simulink model "SF049A_LoaMgr"  (R2013b)
settings: Solver=FixedStepDiscrete  SolverMode=SingleTasking  StartTime=0.0  StopTime=1  FixedStep=0.002  RelTol=1e-3
values from neighbouring files (symbols this model uses):
  CURRMEASLOAMTGTNMASK_CNT_U08 = DataDict.Constant    [SF049A_LoaMgr_DataDict.m]
  IVTRLOAMTGTNMASK_CNT_U08 = DataDict.Constant    [SF049A_LoaMgr_DataDict.m]
  LOAMAXSLEW_ULSPERSEC_F32 = DataDict.Constant    [SF049A_LoaMgr_DataDict.m]
  LoaMgrCurrIvtrMtgtnRate = DataDict.Calibration    [SF049A_LoaMgr_DataDict.m]
  LoaMgrCurrIvtrMtgtnSca = DataDict.Calibration    [SF049A_LoaMgr_DataDict.m]
  LoaMgrCurrIvtrMtgtnScaZeroEna = DataDict.Calibration    [SF049A_LoaMgr_DataDict.m]
  LoaMgrCurrMeasIdptSig0Resp = DataDict.Calibration    [SF049A_LoaMgr_DataDict.m]
  LoaMgrCurrMeasIdptSig1Resp = DataDict.Calibration    [SF049A_LoaMgr_DataDict.m]
  LoaMgrCurrMeasIdptSig2Resp = DataDict.Calibration    [SF049A_LoaMgr_DataDict.m]
  LoaMgrCurrMeasIdptSigFltThd = DataDict.Calibration    [SF049A_LoaMgr_DataDict.m]
  LoaMgrCurrMeasMtgtnRate = DataDict.Calibration    [SF049A_LoaMgr_DataDict.m]
  LoaMgrCurrMeasMtgtnSca = DataDict.Calibration    [SF049A_LoaMgr_DataDict.m]
  LoaMgrCurrMeasMtgtnScaZeroEna = DataDict.Calibration    [SF049A_LoaMgr_DataDict.m]
  LoaMgrFadeOutStRate = DataDict.Calibration    [SF049A_LoaMgr_DataDict.m]
  LoaMgrHwTqIdptSig0NoTqLoaResp = DataDict.Calibration    [SF049A_LoaMgr_DataDict.m]
  LoaMgrHwTqIdptSig1NoTqLoaResp = DataDict.Calibration    [SF049A_LoaMgr_DataDict.m]
  LoaMgrHwTqIdptSig2Resp = DataDict.Calibration    [SF049A_LoaMgr_DataDict.m]
  LoaMgrHwTqIdptSig4Resp = DataDict.Calibration    [SF049A_LoaMgr_DataDict.m]
  LoaMgrHwTqIdptSigFltThd = DataDict.Calibration    [SF049A_LoaMgr_DataDict.m]
  LoaMgrHwTqLoaAvlResp = DataDict.Calibration    [SF049A_LoaMgr_DataDict.m]
  LoaMgrIvtrIdptSig0Resp = DataDict.Calibration    [SF049A_LoaMgr_DataDict.m]
  LoaMgrIvtrIdptSig1Resp = DataDict.Calibration    [SF049A_LoaMgr_DataDict.m]
  LoaMgrIvtrIdptSig2Resp = DataDict.Calibration    [SF049A_LoaMgr_DataDict.m]
  LoaMgrIvtrIdptSigFltThd = DataDict.Calibration    [SF049A_LoaMgr_DataDict.m]
  LoaMgrIvtrMtgtnRate = DataDict.Calibration    [SF049A_LoaMgr_DataDict.m]
  LoaMgrIvtrMtgtnSca = DataDict.Calibration    [SF049A_LoaMgr_DataDict.m]
  LoaMgrIvtrMtgtnScaZeroEna = DataDict.Calibration    [SF049A_LoaMgr_DataDict.m]
  LoaMgrLimdStRate = DataDict.Calibration    [SF049A_LoaMgr_DataDict.m]
  LoaMgrLimdStSca = DataDict.Calibration    [SF049A_LoaMgr_DataDict.m]
  LoaMgrMotAgAvlSnsrlsResp = DataDict.Calibration    [SF049A_LoaMgr_DataDict.m]
  LoaMgrMotAgIdptSig0NoSnsrlsResp = DataDict.Calibration    [SF049A_LoaMgr_DataDict.m]
  LoaMgrMotAgIdptSig1NoSnsrlsResp = DataDict.Calibration    [SF049A_LoaMgr_DataDict.m]
  LoaMgrMotAgIdptSig2Resp = DataDict.Calibration    [SF049A_LoaMgr_DataDict.m]
  LoaMgrMotAgIdptSig3Resp = DataDict.Calibration    [SF049A_LoaMgr_DataDict.m]
  LoaMgrMotAgIdptSigFltThd = DataDict.Calibration    [SF049A_LoaMgr_DataDict.m]
  LoaMgrMotAgMtgtnRate = DataDict.Calibration    [SF049A_LoaMgr_DataDict.m]
  LoaMgrMotAgMtgtnSca = DataDict.Calibration    [SF049A_LoaMgr_DataDict.m]
  LoaMgrMotAgMtgtnScaZeroEna = DataDict.Calibration    [SF049A_LoaMgr_DataDict.m]
  LOASCAONE_ULS_F32 = DataDict.Constant    [SF049A_LoaMgr_DataDict.m]
  LOASCAZERO_ULS_F32 = DataDict.Constant    [SF049A_LoaMgr_DataDict.m]
  LOASTIMDTSHTDWN_CNT_U08 = DataDict.Constant    [SF049A_LoaMgr_DataDict.m]
  LOASTNORM_CNT_U08 = DataDict.Constant    [SF049A_LoaMgr_DataDict.m]
  LOASTSWMTGTN_CNT_U08 = DataDict.Constant    [SF049A_LoaMgr_DataDict.m]
  MAXCURRMEASIDPTSIGALLWD_CNT_U08 = DataDict.Constant    [SF049A_LoaMgr_DataDict.m]
  MAXHWTQIDPTSIGALLWD_CNT_U08 = DataDict.Constant    [SF049A_LoaMgr_DataDict.m]
  MAXIVTRIDPTSIGALLWD_CNT_U08 = DataDict.Constant    [SF049A_LoaMgr_DataDict.m]
  MAXMOTAGMECLIDPTSIGALLWD_CNT_U08 = DataDict.Constant    [SF049A_LoaMgr_DataDict.m]
  NODEBSTEP_CNT_U16 = DataDict.Constant    [SF049A_LoaMgr_DataDict.m]
undefined symbols (not defined in the file or in its folder): LoaSt1, NtcNr1, NtcSts1, SigQlfr1
libraries: simulink x43, NxtrMin x4, NxtrMax x4, NxtrLim x2
(part 2 of 8)

== system SF049A_LoaMgr/ISO Fault Debounce/DiagMgr/NTCSTS_PREPASSD ==
  EA : Inport
  DS : Inport  Port=2
  TS : Inport  Port=3
  Qlf : Inport  Port=4
  Action Port : ActionPort  ActionType=case
  CopyRight2 : Subsystem  Description=|  mask(Copyright Information){none=on}
      | Copyright info block.                                               
      |                                                                     
      | Place copyright information at the top of every subsystem in design.
      mask prompts: none "No parameters"
      mask help: Place copyright information at the top of every subsystem in design.
      mask Display:
      | NxtrConf = 'Nexteer Confidential';
      | 
      | sys = bdroot; %handle for the current model ("system")
      | first = get_param(sys,'Created');
      | first = first(end-3:end);  %year is last four digits
      | 
      | last = get_param(sys,'LastModifiedDate');
      | if isempty(last)
      |     last = datestr(now,'yyyy');
      | else
      |     last = last(end-3:end);
      | end
      | 
      | if strcmp(first,last)
      |     fprintf('%s -- Copyright %s Nexteer',NxtrConf,first)
      | else
      |     fprintf('%s -- %s%s- %s Nexteer',NxtrConf,char(169),first,last)
      | end
  If : If  NumInputs=2  IfExpression=u1 <= u2
  If Action Subsystem : Subsystem  TreatAsAtomicUnit=on
  If Action Subsystem1 : Subsystem  TreatAsAtomicUnit=on
  Merge : Merge
  Merge1 : Merge
  QlfPassd : Constant  Value=SigQlfr1.SIGQLFR_PASSD  OutDataTypeStr=Enum: SigQlfr1
  Sum : Sum  Inputs=|+-
  Unary Minus : UnaryMinus
  EAo : Outport
  Qlfo : Outport  Port=2
  wires:
  EA/1 -> Sum/1
  DS/1 -> Sum/2
  Sum/1 -> If Action Subsystem1/1(In1), If/1
  TS/1 -> [Threshold], If/2
  If/1 -> If Action Subsystem/Action
  Unary Minus/1 -> If Action Subsystem/1(In1)
  If Action Subsystem/1(Out1) -> Merge/1
  If Action Subsystem1/1(Out1) -> Merge/2
  Merge/1 -> EAo/1
  If Action Subsystem/2(Out2) -> Merge1/1
  If Action Subsystem1/2(Out2) -> Merge1/2
  Merge1/1 -> Qlfo/1
  QlfPassd/1 -> If Action Subsystem/2(In2)
  Qlf/1 -> If Action Subsystem1/2(In2)
  If/2 -> If Action Subsystem1/Action
  [Threshold] -> Unary Minus/1

== system SF049A_LoaMgr/ISO Fault Debounce/DiagMgr/Set Latch ==
  In1 : Inport
  Action Port : ActionPort  ActionType=then
  Out1 : Outport
  wires:
  In1/1 -> Out1/1

== system SF049A_LoaMgr/LoaMgr/LoaMgrInit1/CopyRight2 ==

== system SF049A_LoaMgr/LoaMgr/LoaMgrInit1/NTC_Fault1 ==
  NtcNr : Inport
  NtcStInfo : Inport  Port=2
  NtcSts : Inport  Port=3
  DebStep : Inport  Port=4
  SetNtcSts : Subsystem  RequirementInfo={} %GIDa_23fdb935_d0cd_490e_ba1d_400dad3b5aaf  TreatAsAtomicUnit=on
      settings: RTWSystemCode=Inline
  wires:
  NtcNr/1 -> SetNtcSts/1(NtcNr)  "NtcNr"
  NtcSts/1 -> SetNtcSts/3(NtcSts)
  DebStep/1 -> SetNtcSts/4(DebStep)
  NtcStInfo/1 -> SetNtcSts/2(NtcStInfo)

== system SF049A_LoaMgr/LoaMgr/LoaMgrInit1/NTC_Fault2 ==
  NtcNr : Inport
  NtcStInfo : Inport  Port=2
  NtcSts : Inport  Port=3
  DebStep : Inport  Port=4
  SetNtcSts : Subsystem  RequirementInfo={} %GIDa_89eb5662_1adb_446a_ae4b_e7f3c6b102b6  TreatAsAtomicUnit=on
      settings: RTWSystemCode=Inline
  wires:
  NtcStInfo/1 -> SetNtcSts/2(NtcStInfo)
  DebStep/1 -> SetNtcSts/4(DebStep)
  NtcSts/1 -> SetNtcSts/3(NtcSts)
  NtcNr/1 -> SetNtcSts/1(NtcNr)  "NtcNr"

== system SF049A_LoaMgr/LoaMgr/LoaMgrInit1/NTC_Fault3 ==
  NtcNr : Inport
  NtcStInfo : Inport  Port=2
  NtcSts : Inport  Port=3
  DebStep : Inport  Port=4
  SetNtcSts : Subsystem  RequirementInfo={} %GIDa_2736ae0d_ecf6_416e_8429_36e35a164155  TreatAsAtomicUnit=on
      settings: RTWSystemCode=Inline
  wires:
  NtcStInfo/1 -> SetNtcSts/2(NtcStInfo)
  DebStep/1 -> SetNtcSts/4(DebStep)
  NtcSts/1 -> SetNtcSts/3(NtcSts)
  NtcNr/1 -> SetNtcSts/1(NtcNr)  "NtcNr"

== system SF049A_LoaMgr/LoaMgr/LoaMgrInit1/NTC_Fault4 ==
  NtcNr : Inport
  NtcStInfo : Inport  Port=2
  NtcSts : Inport  Port=3
  DebStep : Inport  Port=4
  SetNtcSts : Subsystem  RequirementInfo={} %GIDa_c84246ca_06da_45c0_bfee_0800e0212aeb  TreatAsAtomicUnit=on
      settings: RTWSystemCode=Inline
  wires:
  NtcNr/1 -> SetNtcSts/1(NtcNr)  "NtcNr"
  NtcSts/1 -> SetNtcSts/3(NtcSts)
  DebStep/1 -> SetNtcSts/4(DebStep)
  NtcStInfo/1 -> SetNtcSts/2(NtcStInfo)

== system SF049A_LoaMgr/LoaMgr/LoaMgrInit1/NTC_Fault5 ==
  NtcNr : Inport
  NtcStInfo : Inport  Port=2
  NtcSts : Inport  Port=3
  DebStep : Inport  Port=4
  SetNtcSts : Subsystem  RequirementInfo={} %GIDa_5e8c2de6_0cb9_44b1_8719_e4221f2f855f  TreatAsAtomicUnit=on
      settings: RTWSystemCode=Inline
  wires:
  NtcStInfo/1 -> SetNtcSts/2(NtcStInfo)
  DebStep/1 -> SetNtcSts/4(DebStep)
  NtcSts/1 -> SetNtcSts/3(NtcSts)
  NtcNr/1 -> SetNtcSts/1(NtcNr)  "NtcNr"

== system SF049A_LoaMgr/LoaMgr/LoaMgrInit1/NTC_Fault6 ==
  NtcNr : Inport
  NtcStInfo : Inport  Port=2
  NtcSts : Inport  Port=3
  DebStep : Inport  Port=4
  SetNtcSts : Subsystem  RequirementInfo={} %GIDa_1fd4e5c0_5e97_4c72_b752_8c7dcd130455  TreatAsAtomicUnit=on
      settings: RTWSystemCode=Inline
  wires:
  NtcStInfo/1 -> SetNtcSts/2(NtcStInfo)
  DebStep/1 -> SetNtcSts/4(DebStep)
  NtcSts/1 -> SetNtcSts/3(NtcSts)
  NtcNr/1 -> SetNtcSts/1(NtcNr)  "NtcNr"

== system SF049A_LoaMgr/LoaMgr/LoaMgrPer1/Arbitrate_Responses ==
  note: Individual responses can set boolean flags to true to direct downstream functions.
      | The combination of individual responses generates its own "multiple mitigation response".
      | The final LoaState response will be the worst case of individual and "multiple mitigation" responses.
  RespMux : Inport
  CntSwBasdMtgtn : Subsystem
  CopyRight2 : Subsystem  Description=|  mask(Copyright Information){none=on}
      | Copyright info block.                                               
      |                                                                     
      | Place copyright information at the top of every subsystem in design.
      mask prompts: none "No parameters"
      mask help: Place copyright information at the top of every subsystem in design.
      mask Display:
      | NxtrConf = 'Nexteer Confidential';
      | 
      | sys = bdroot; %handle for the current model ("system")
      | first = get_param(sys,'Created');
      | first = first(end-3:end);  %year is last four digits
      | 
      | last = get_param(sys,'LastModifiedDate');
      | if isempty(last)
      |     last = datestr(now,'yyyy');
      | else
      |     last = last(end-3:end);
      | end
      | 
      | if strcmp(first,last)
      |     fprintf('%s -- Copyright %s Nexteer',NxtrConf,first)
      | else
      |     fprintf('%s -- %s%s- %s Nexteer',NxtrConf,char(169),first,last)
      | end
  Demux : Demux
  Demux1 : Demux
  Mux : Mux
  SelFinalResp : Subsystem
  LoaState : Outport  RequirementInfo="{'linktype_rmi_doors' '0000bab3 (/E-STEER Core/SubSystem Specifications/Application Functions/SF049A Loss of Assist Manager)' '#SF049A_84' 'true' 'REQ:  SF049A_84' '' } %GIDa_2917bb2b_4bd4_4079_ac09_4ef15e442a03"
  SwMtgtnEnMux : Outport  Port=2
  wires:
  Demux/1 -> CntSwBasdMtgtn/1(HwTqResp)
  Demux/2 -> CntSwBasdMtgtn/2(MotAgResp)
  Demux/3 -> CntSwBasdMtgtn/3(CurrMeasResp)
  Demux/4 -> CntSwBasdMtgtn/4(IvtrResp)
  CntSwBasdMtgtn/1(HwTqLoaMtgtnEna) -> Mux/1  "HwTqLoaMtgtnEna"
  CntSwBasdMtgtn/2(MotAgLoaMtgtnEna) -> Mux/2  "MotAgLoaMtgtnEna"
  CntSwBasdMtgtn/3(CurrMeasLoaMtgtnEna) -> Mux/3  "CurrMeasLoaMtgtnEna"
  CntSwBasdMtgtn/4(IvtrLoaMtgtnEna) -> Mux/4  "IvtrLoaMtgtnEna"
  Mux/1 -> SwMtgtnEnMux/1
  CntSwBasdMtgtn/5(MultiMtgtnResp) -> SelFinalResp/1(MultiMtgtnResp)
  RespMux/1 -> Demux1/1, Demux/1
  Demux1/1 -> SelFinalResp/2(HwTqResp)
  Demux1/2 -> SelFinalResp/3(MotAgResp)
  Demux1/3 -> SelFinalResp/4(CurrMeasResp)
  Demux1/4 -> SelFinalResp/5(IvtrResp)
  SelFinalResp/1(LoaSt) -> LoaState/1

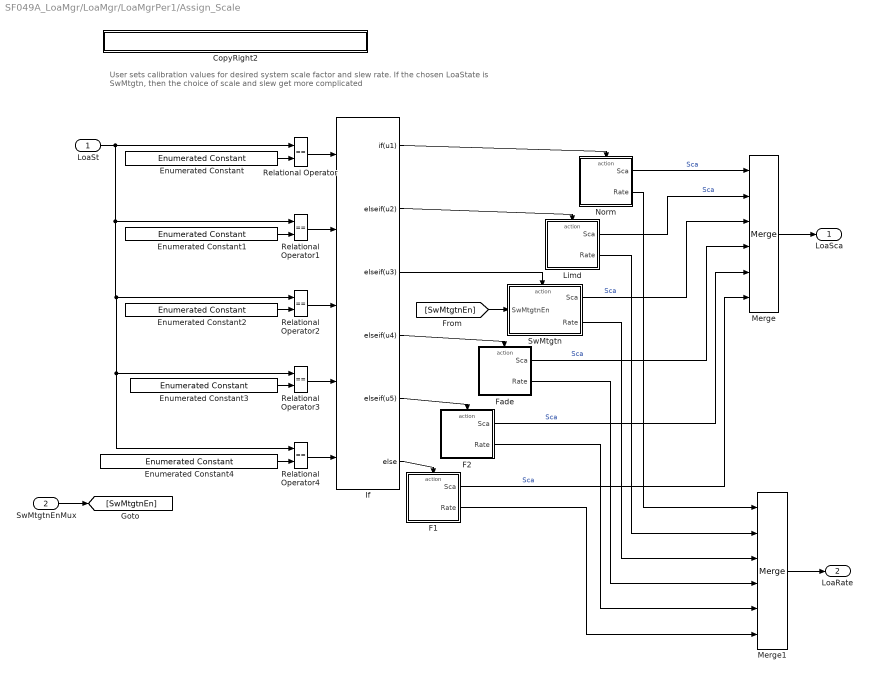
== system SF049A_LoaMgr/LoaMgr/LoaMgrPer1/Assign_Scale ==
  note: User sets calibration values for desired system scale factor and slew rate.  If the chosen LoaState is SwMtgtn, then the choice of
      | scale and slew get more complicated
  LoaSt : Inport  RequirementInfo="{'linktype_rmi_doors' '0000bab3 (/E-STEER Core/SubSystem Specifications/Application Functions/SF049A Loss of Assist Manager)' '#SF049A_93' 'true' 'REQ:  SF049A_93' '' ; 'linktype_rmi_doors' '0000bab3 (/E-STEER Core/SubSystem Specifications/Application Functions/SF049A Loss of Assist Manager)' '#SF049A_94' 'true' 'REQ:  SF049A_94' '' ; 'linktype_rmi_doors' '0000bab3 (/E-STEER Core/SubSystem Specifications/Application Functions/SF049A Loss of Assist Manager)' '#SF049A_95' 'true' 'REQ:  SF049A_95' '' ; 'linktype_rmi_doors' '0000bab3 (/E-STEER Core/SubSystem Specifications/Application Functions/SF049A Loss of Assist Manager)' '#SF049A_96' 'true' 'REQ:  SF049A_96' '' ; 'linktype_rmi_doors' '0000bab3 (/E-STEER Core/SubSystem Specifications/Application Functions/SF049A Loss of Assist Manager)' '#SF049A_97' 'true' 'REQ:  SF049A_97' '' ; 'linktype_rmi_doors' '0000bab3 (/E-STEER Core/SubSystem Specifications/Application Functions/SF049A Loss of Assist Manager)' '#SF049A_100' 'true' 'REQ:  SF049A_100' '' } %GIDa_3e7875f7_b2dd_4b11_87a2_7c0344e13c7b"
  SwMtgtnEnMux : Inport  RequirementInfo="{'linktype_rmi_doors' '0000bab3 (/E-STEER Core/SubSystem Specifications/Application Functions/SF049A Loss of Assist Manager)' '#SF049A_99' 'true' 'REQ:  SF049A_99' '' ; 'linktype_rmi_doors' '0000bab3 (/E-STEER Core/SubSystem Specifications/Application Functions/SF049A Loss of Assist Manager)' '#SF049A_100' 'true' 'REQ:  SF049A_100' '' } %GIDa_9818a3a5_64db_45b2_8dab_2de682de8c50"  Port=2
  CopyRight2 : Subsystem  Description=|  mask(Copyright Information){none=on}
      | Copyright info block.                                               
      |                                                                     
      | Place copyright information at the top of every subsystem in design.
      mask prompts: none "No parameters"
      mask help: Place copyright information at the top of every subsystem in design.
      mask Display:
      | NxtrConf = 'Nexteer Confidential';
      | 
      | sys = bdroot; %handle for the current model ("system")
      | first = get_param(sys,'Created');
      | first = first(end-3:end);  %year is last four digits
      | 
      | last = get_param(sys,'LastModifiedDate');
      | if isempty(last)
      |     last = datestr(now,'yyyy');
      | else
      |     last = last(end-3:end);
      | end
      | 
      | if strcmp(first,last)
      |     fprintf('%s -- Copyright %s Nexteer',NxtrConf,first)
      | else
      |     fprintf('%s -- %s%s- %s Nexteer',NxtrConf,char(169),first,last)
      | end
  Enumerated Constant : simulink/Sources/Enumerated Constant  RequirementInfo="{'linktype_rmi_doors' '0000bab3 (/E-STEER Core/SubSystem Specifications/Application Functions/SF049A Loss of Assist Manager)' '#SF049A_93' 'true' 'REQ:  SF049A_93' '' } %GIDa_f27a0b99_a290_4ea5_abd7_4a8bd3123567"  OutDataTypeStr=Enum: LoaSt1  Value=LoaSt1.LOAST_NORM  SampleTime=inf
  Enumerated Constant1 : simulink/Sources/Enumerated Constant  RequirementInfo="{'linktype_rmi_doors' '0000bab3 (/E-STEER Core/SubSystem Specifications/Application Functions/SF049A Loss of Assist Manager)' '#SF049A_94' 'true' 'REQ:  SF049A_94' '' } %GIDa_d920381e_876a_4e76_93ae_b2656d59d1b0"  OutDataTypeStr=Enum: LoaSt1  Value=LoaSt1.LOAST_LIMD  SampleTime=inf
  Enumerated Constant2 : simulink/Sources/Enumerated Constant  RequirementInfo="{'linktype_rmi_doors' '0000bab3 (/E-STEER Core/SubSystem Specifications/Application Functions/SF049A Loss of Assist Manager)' '#SF049A_99' 'true' 'REQ:  SF049A_99' '' ; 'linktype_rmi_doors' '0000bab3 (/E-STEER Core/SubSystem Specifications/Application Functions/SF049A Loss of Assist Manager)' '#SF049A_100' 'true' 'REQ:  SF049A_100' '' } %GIDa_83a64fdd_b2aa_4bd7_b652_9878089e09b4"  OutDataTypeStr=Enum: LoaSt1  Value=LoaSt1.LOAST_SWBASDMTGTN  SampleTime=inf
  Enumerated Constant3 : simulink/Sources/Enumerated Constant  RequirementInfo="{'linktype_rmi_doors' '0000bab3 (/E-STEER Core/SubSystem Specifications/Application Functions/SF049A Loss of Assist Manager)' '#SF049A_95' 'true' 'REQ:  SF049A_95' '' } %GIDa_647ea362_d5ca_4b6a_9517_1cd75c76e2d9"  OutDataTypeStr=Enum: LoaSt1  Value=LoaSt1.LOAST_FADEOUT  SampleTime=inf
  Enumerated Constant4 : simulink/Sources/Enumerated Constant  RequirementInfo="{'linktype_rmi_doors' '0000bab3 (/E-STEER Core/SubSystem Specifications/Application Functions/SF049A Loss of Assist Manager)' '#SF049A_96' 'true' 'REQ:  SF049A_96' '' } %GIDa_cd78f97b_5efc_4e4a_8ad5_30890b04384b"  OutDataTypeStr=Enum: LoaSt1  Value=LoaSt1.LOAST_CTRLDSHTDWNREQD  SampleTime=inf
  F1 : Subsystem  RequirementInfo="{'linktype_rmi_doors' '0000bab3 (/E-STEER Core/SubSystem Specifications/Application Functions/SF049A Loss of Assist Manager)' '#SF049A_97' 'true' 'REQ:  SF049A_97' '' } %GIDa_e1aaa04d_b9cf_4590_9790_e96624afa4aa"  TreatAsAtomicUnit=on
      settings: RTWSystemCode=Inline
  F2 : Subsystem  RequirementInfo="{'linktype_rmi_doors' '0000bab3 (/E-STEER Core/SubSystem Specifications/Application Functions/SF049A Loss of Assist Manager)' '#SF049A_96' 'true' 'REQ:  SF049A_96' '' } %GIDa_1938d1a4_6ea2_4bb3_af5e_d31a0fe8b378"  TreatAsAtomicUnit=on
      settings: RTWSystemCode=Inline
  Fade : Subsystem  RequirementInfo="{'linktype_rmi_doors' '0000bab3 (/E-STEER Core/SubSystem Specifications/Application Functions/SF049A Loss of Assist Manager)' '#SF049A_95' 'true' 'REQ:  SF049A_95' '' } %GIDa_5c4662ce_ee53_4f4f_ae03_f1d5fbfaeef4"  TreatAsAtomicUnit=on
      settings: RTWSystemCode=Inline
  If : If  RequirementInfo="{'linktype_rmi_doors' '0000bab3 (/E-STEER Core/SubSystem Specifications/Application Functions/SF049A Loss of Assist Manager)' '#SF049A_93' 'true' 'REQ:  SF049A_93' '' ; 'linktype_rmi_doors' '0000bab3 (/E-STEER Core/SubSystem Specifications/Application Functions/SF049A Loss of Assist Manager)' '#SF049A_94' 'true' 'REQ:  SF049A_94' '' ; 'linktype_rmi_doors' '0000bab3 (/E-STEER Core/SubSystem Specifications/Application Functions/SF049A Loss of Assist Manager)' '#SF049A_95' 'true' 'REQ:  SF049A_95' '' ; 'linktype_rmi_doors' '0000bab3 (/E-STEER Core/SubSystem Specifications/Application Functions/SF049A Loss of Assist Manager)' '#SF049A_96' 'true' 'REQ:  SF049A_96' '' ; 'linktype_rmi_doors' '0000bab3 (/E-STEER Core/SubSystem Specifications/Application Functions/SF049A Loss of Assist Manager)' '#SF049A_97' 'true' 'REQ:  SF049A_97' '' ; 'linktype_rmi_doors' '0000bab3 (/E-STEER Core/SubSystem Specifications/Application Functions/SF049A Loss of Assist Manager)' '#SF049A_99' 'true' 'REQ:  SF049A_99' '' ; 'linktype_rmi_doors' '0000bab3 (/E-STEER Core/SubSystem Specifications/Application Functions/SF049A Loss of Assist Manager)' '#SF049A_100' 'true' 'REQ:  SF049A_100' '' } %GIDa_5c51bdba_2274_48ad_8412_9716f3180cc7"  NumInputs=5  IfExpression=u1  ElseIfExpressions=u2, u3,u4,u5
  Limd : Subsystem  RequirementInfo="{'linktype_rmi_doors' '0000bab3 (/E-STEER Core/SubSystem Specifications/Application Functions/SF049A Loss of Assist Manager)' '#SF049A_94' 'true' 'REQ:  SF049A_94' '' } %GIDa_f0a5710c_890a_4ef1_b79a_7c37771acf89"  TreatAsAtomicUnit=on
      settings: RTWSystemCode=Inline
  Merge : Merge  RequirementInfo="{'linktype_rmi_doors' '0000bab3 (/E-STEER Core/SubSystem Specifications/Application Functions/SF049A Loss of Assist Manager)' '#SF049A_93' 'true' 'REQ:  SF049A_93' '' ; 'linktype_rmi_doors' '0000bab3 (/E-STEER Core/SubSystem Specifications/Application Functions/SF049A Loss of Assist Manager)' '#SF049A_94' 'true' 'REQ:  SF049A_94' '' ; 'linktype_rmi_doors' '0000bab3 (/E-STEER Core/SubSystem Specifications/Application Functions/SF049A Loss of Assist Manager)' '#SF049A_95' 'true' 'REQ:  SF049A_95' '' ; 'linktype_rmi_doors' '0000bab3 (/E-STEER Core/SubSystem Specifications/Application Functions/SF049A Loss of Assist Manager)' '#SF049A_96' 'true' 'REQ:  SF049A_96' '' ; 'linktype_rmi_doors' '0000bab3 (/E-STEER Core/SubSystem Specifications/Application Functions/SF049A Loss of Assist Manager)' '#SF049A_97' 'true' 'REQ:  SF049A_97' '' ; 'linktype_rmi_doors' '0000bab3 (/E-STEER Core/SubSystem Specifications/Application Functions/SF049A Loss of Assist Manager)' '#SF049A_99' 'true' 'REQ:  SF049A_99' '' ; 'linktype_rmi_doors' '0000bab3 (/E-STEER Core/SubSystem Specifications/Application Functions/SF049A Loss of Assist Manager)' '#SF049A_100' 'true' 'REQ:  SF049A_100' '' } %GIDa_3b299f34_e795_470f_ac90_16d0d3d510be"  Inputs=6
  Merge1 : Merge  RequirementInfo="{'linktype_rmi_doors' '0000bab3 (/E-STEER Core/SubSystem Specifications/Application Functions/SF049A Loss of Assist Manager)' '#SF049A_93' 'true' 'REQ:  SF049A_93' '' ; 'linktype_rmi_doors' '0000bab3 (/E-STEER Core/SubSystem Specifications/Application Functions/SF049A Loss of Assist Manager)' '#SF049A_94' 'true' 'REQ:  SF049A_94' '' ; 'linktype_rmi_doors' '0000bab3 (/E-STEER Core/SubSystem Specifications/Application Functions/SF049A Loss of Assist Manager)' '#SF049A_95' 'true' 'REQ:  SF049A_95' '' ; 'linktype_rmi_doors' '0000bab3 (/E-STEER Core/SubSystem Specifications/Application Functions/SF049A Loss of Assist Manager)' '#SF049A_96' 'true' 'REQ:  SF049A_96' '' ; 'linktype_rmi_doors' '0000bab3 (/E-STEER Core/SubSystem Specifications/Application Functions/SF049A Loss of Assist Manager)' '#SF049A_97' 'true' 'REQ:  SF049A_97' '' ; 'linktype_rmi_doors' '0000bab3 (/E-STEER Core/SubSystem Specifications/Application Functions/SF049A Loss of Assist Manager)' '#SF049A_99' 'true' 'REQ:  SF049A_99' '' ; 'linktype_rmi_doors' '0000bab3 (/E-STEER Core/SubSystem Specifications/Application Functions/SF049A Loss of Assist Manager)' '#SF049A_100' 'true' 'REQ:  SF049A_100' '' } %GIDa_74c15a35_1fbd_4169_b897_3cf740b201ea"  Inputs=6
  Norm : Subsystem  RequirementInfo="{'linktype_rmi_doors' '0000bab3 (/E-STEER Core/SubSystem Specifications/Application Functions/SF049A Loss of Assist Manager)' '#SF049A_93' 'true' 'REQ:  SF049A_93' '' } %GIDa_c9df33ca_5dd7_489e_a91a_aa4b767aa5db"  TreatAsAtomicUnit=on
      settings: RTWSystemCode=Inline
  Relational Operator : RelationalOperator  RequirementInfo="{'linktype_rmi_doors' '0000bab3 (/E-STEER Core/SubSystem Specifications/Application Functions/SF049A Loss of Assist Manager)' '#SF049A_93' 'true' 'REQ:  SF049A_93' '' } %GIDa_da08ce41_39bd_4e01_b620_6f9860489864"  Operator===  OutDataTypeStr=boolean
  Relational Operator1 : RelationalOperator  RequirementInfo="{'linktype_rmi_doors' '0000bab3 (/E-STEER Core/SubSystem Specifications/Application Functions/SF049A Loss of Assist Manager)' '#SF049A_94' 'true' 'REQ:  SF049A_94' '' } %GIDa_10d94627_2d94_4d9c_8055_2d3addac56cd"  Operator===  OutDataTypeStr=boolean
  Relational Operator2 : RelationalOperator  RequirementInfo="{'linktype_rmi_doors' '0000bab3 (/E-STEER Core/SubSystem Specifications/Application Functions/SF049A Loss of Assist Manager)' '#SF049A_99' 'true' 'REQ:  SF049A_99' '' ; 'linktype_rmi_doors' '0000bab3 (/E-STEER Core/SubSystem Specifications/Application Functions/SF049A Loss of Assist Manager)' '#SF049A_100' 'true' 'REQ:  SF049A_100' '' } %GIDa_6fb469fc_d1b3_4ed9_bf7f_ce037c3366d3"  Operator===  OutDataTypeStr=boolean
  Relational Operator3 : RelationalOperator  RequirementInfo="{'linktype_rmi_doors' '0000bab3 (/E-STEER Core/SubSystem Specifications/Application Functions/SF049A Loss of Assist Manager)' '#SF049A_95' 'true' 'REQ:  SF049A_95' '' } %GIDa_85f97dac_396b_438a_bfaa_297eb3998244"  Operator===  OutDataTypeStr=boolean
  Relational Operator4 : RelationalOperator  RequirementInfo="{'linktype_rmi_doors' '0000bab3 (/E-STEER Core/SubSystem Specifications/Application Functions/SF049A Loss of Assist Manager)' '#SF049A_96' 'true' 'REQ:  SF049A_96' '' } %GIDa_ea11fa20_b626_4bfa_a544_554563d25da6"  Operator===  OutDataTypeStr=boolean
  SwMtgtn : Subsystem  RequirementInfo="{'linktype_rmi_doors' '0000bab3 (/E-STEER Core/SubSystem Specifications/Application Functions/SF049A Loss of Assist Manager)' '#SF049A_99' 'true' 'REQ:  SF049A_99' '' ; 'linktype_rmi_doors' '0000bab3 (/E-STEER Core/SubSystem Specifications/Application Functions/SF049A Loss of Assist Manager)' '#SF049A_100' 'true' 'REQ:  SF049A_100' '' } %GIDa_0f2bff9a_81bf_40ef_b624_524280b34e28"  TreatAsAtomicUnit=on
      settings: RTWSystemCode=Inline
  LoaSca : Outport  RequirementInfo="{'linktype_rmi_doors' '0000bab3 (/E-STEER Core/SubSystem Specifications/Application Functions/SF049A Loss of Assist Manager)' '#SF049A_93' 'true' 'REQ:  SF049A_93' '' ; 'linktype_rmi_doors' '0000bab3 (/E-STEER Core/SubSystem Specifications/Application Functions/SF049A Loss of Assist Manager)' '#SF049A_94' 'true' 'REQ:  SF049A_94' '' ; 'linktype_rmi_doors' '0000bab3 (/E-STEER Core/SubSystem Specifications/Application Functions/SF049A Loss of Assist Manager)' '#SF049A_95' 'true' 'REQ:  SF049A_95' '' ; 'linktype_rmi_doors' '0000bab3 (/E-STEER Core/SubSystem Specifications/Application Functions/SF049A Loss of Assist Manager)' '#SF049A_96' 'true' 'REQ:  SF049A_96' '' ; 'linktype_rmi_doors' '0000bab3 (/E-STEER Core/SubSystem Specifications/Application Functions/SF049A Loss of Assist Manager)' '#SF049A_97' 'true' 'REQ:  SF049A_97' '' ; 'linktype_rmi_doors' '0000bab3 (/E-STEER Core/SubSystem Specifications/Application Functions/SF049A Loss of Assist Manager)' '#SF049A_99' 'true' 'REQ:  SF049A_99' '' ; 'linktype_rmi_doors' '0000bab3 (/E-STEER Core/SubSystem Specifications/Application Functions/SF049A Loss of Assist Manager)' '#SF049A_100' 'true' 'REQ:  SF049A_100' '' } %GIDa_169a2149_2e31_4d28_bbf1_074d98108588"
  LoaRate : Outport  RequirementInfo="{'linktype_rmi_doors' '0000bab3 (/E-STEER Core/SubSystem Specifications/Application Functions/SF049A Loss of Assist Manager)' '#SF049A_93' 'true' 'REQ:  SF049A_93' '' ; 'linktype_rmi_doors' '0000bab3 (/E-STEER Core/SubSystem Specifications/Application Functions/SF049A Loss of Assist Manager)' '#SF049A_94' 'true' 'REQ:  SF049A_94' '' ; 'linktype_rmi_doors' '0000bab3 (/E-STEER Core/SubSystem Specifications/Application Functions/SF049A Loss of Assist Manager)' '#SF049A_95' 'true' 'REQ:  SF049A_95' '' ; 'linktype_rmi_doors' '0000bab3 (/E-STEER Core/SubSystem Specifications/Application Functions/SF049A Loss of Assist Manager)' '#SF049A_96' 'true' 'REQ:  SF049A_96' '' ; 'linktype_rmi_doors' '0000bab3 (/E-STEER Core/SubSystem Specifications/Application Functions/SF049A Loss of Assist Manager)' '#SF049A_97' 'true' 'REQ:  SF049A_97' '' ; 'linktype_rmi_doors' '0000bab3 (/E-STEER Core/SubSystem Specifications/Application Functions/SF049A Loss of Assist Manager)' '#SF049A_99' 'true' 'REQ:  SF049A_99' '' ; 'linktype_rmi_doors' '0000bab3 (/E-STEER Core/SubSystem Specifications/Application Functions/SF049A Loss of Assist Manager)' '#SF049A_100' 'true' 'REQ:  SF049A_100' '' } %GIDa_8cb2e7f7_efc3_4bfe_b724_767c9179be15"  Port=2
  wires:
  Enumerated Constant/1 -> Relational Operator/2
  Enumerated Constant1/1 -> Relational Operator1/2
  Enumerated Constant2/1 -> Relational Operator2/2
  Enumerated Constant3/1 -> Relational Operator3/2
  LoaSt/1 -> Relational Operator4/1, Relational Operator3/1, Relational Operator2/1, Relational Operator1/1, Relational Operator/1
  Enumerated Constant4/1 -> Relational Operator4/2
  Relational Operator/1 -> If/1
  Relational Operator1/1 -> If/2
  Relational Operator2/1 -> If/3
  Relational Operator3/1 -> If/4
  Relational Operator4/1 -> If/5
  If/1 -> Norm/Action
  If/2 -> Limd/Action
  If/3 -> SwMtgtn/Action
  If/4 -> Fade/Action
  If/5 -> F2/Action
  If/6 -> F1/Action
  Norm/1(Sca) -> Merge/1  "Sca"
  Limd/1(Sca) -> Merge/2  "Sca"
  Fade/1(Sca) -> Merge/4  "Sca"
  F2/1(Sca) -> Merge/5  "Sca"
  F1/1(Sca) -> Merge/6  "Sca"
  Merge/1 -> LoaSca/1
  Norm/2(Rate) -> Merge1/1
  Limd/2(Rate) -> Merge1/2
  Fade/2(Rate) -> Merge1/4
  F2/2(Rate) -> Merge1/5
  F1/2(Rate) -> Merge1/6
  Merge1/1 -> LoaRate/1
  SwMtgtnEnMux/1 -> [SwMtgtnEn]
  [SwMtgtnEn] -> SwMtgtn/1(SwMtgtnEn)
  SwMtgtn/1(Sca) -> Merge/3  "Sca"
  SwMtgtn/2(Rate) -> Merge1/3

== system SF049A_LoaMgr/LoaMgr/LoaMgrPer1/Calc_Ivtr_State ==
  note: Nexter coding standards prevent the casting of boolean signals to other datatypes.
      | If that rule did not exist, this logic would use convert blocks to cast each boolean
      | to uint8, then add them up.
  Ivtr1Inactv : Inport  RequirementInfo="{'linktype_rmi_doors' '0000bab3 (/E-STEER Core/SubSystem Specifications/Application Functions/SF049A Loss of Assist Manager)' '#SF049A_183' 'true' 'REQ:  SF049A_183' '' } %GIDa_de6ec2ea_e682_4d17_b4f6_aabeca528bd3"
  Ivtr2Inactv : Inport  RequirementInfo="{'linktype_rmi_doors' '0000bab3 (/E-STEER Core/SubSystem Specifications/Application Functions/SF049A Loss of Assist Manager)' '#SF049A_183' 'true' 'REQ:  SF049A_183' '' } %GIDa_968df205_4920_4db1_82fc_3b23eb8eeb61"  Port=2
  " " : Merge  RequirementInfo="{'linktype_rmi_doors' '0000bab3 (/E-STEER Core/SubSystem Specifications/Application Functions/SF049A Loss of Assist Manager)' '#SF049A_183' 'true' 'REQ:  SF049A_183' '' } %GIDa_6e820a2a_9d7d_4387_81a9_e3b6b43a99ee"
  " 1" : Merge  RequirementInfo="{'linktype_rmi_doors' '0000bab3 (/E-STEER Core/SubSystem Specifications/Application Functions/SF049A Loss of Assist Manager)' '#SF049A_183' 'true' 'REQ:  SF049A_183' '' } %GIDa_4be40db0_e2f0_494d_962c_150a10a22e37"
  Add1 : Sum  RequirementInfo="{'linktype_rmi_doors' '0000bab3 (/E-STEER Core/SubSystem Specifications/Application Functions/SF049A Loss of Assist Manager)' '#SF049A_183' 'true' 'REQ:  SF049A_183' '' } %GIDa_6635589d_766f_4912_9afd_5eff77041ff3"
  Constant1 : Constant  RequirementInfo="{'linktype_rmi_doors' '0000bab3 (/E-STEER Core/SubSystem Specifications/Application Functions/SF049A Loss of Assist Manager)' '#SF049A_183' 'true' 'REQ:  SF049A_183' '' } %GIDa_41bc2e65_c215_4d13_87d4_1d9f310de0af"  OutDataTypeStr=uint8
      settings: AttributesFormatString=%<OutDataTypeStr>
  Constant2 : Constant  RequirementInfo="{'linktype_rmi_doors' '0000bab3 (/E-STEER Core/SubSystem Specifications/Application Functions/SF049A Loss of Assist Manager)' '#SF049A_183' 'true' 'REQ:  SF049A_183' '' } %GIDa_12d9b86f_40e2_490f_b7b6_b5286bb30cc6"  Value=0  OutDataTypeStr=uint8
      settings: AttributesFormatString=%<OutDataTypeStr>
  Constant4 : Constant  RequirementInfo="{'linktype_rmi_doors' '0000bab3 (/E-STEER Core/SubSystem Specifications/Application Functions/SF049A Loss of Assist Manager)' '#SF049A_183' 'true' 'REQ:  SF049A_183' '' } %GIDa_91ec947b_8597_46f0_9f25_34857e4f337d"  Value=0  OutDataTypeStr=uint8
      settings: AttributesFormatString=%<OutDataTypeStr>
  Constant6 : Constant  RequirementInfo="{'linktype_rmi_doors' '0000bab3 (/E-STEER Core/SubSystem Specifications/Application Functions/SF049A Loss of Assist Manager)' '#SF049A_183' 'true' 'REQ:  SF049A_183' '' } %GIDa_cebea097_c2b2_4a90_91e2_d089833dbd9f"  OutDataTypeStr=uint8
      settings: AttributesFormatString=%<OutDataTypeStr>
  CopyRight2 : Subsystem  Description=|  mask(Copyright Information){none=on}
      | Copyright info block.                                               
      |                                                                     
      | Place copyright information at the top of every subsystem in design.
      mask prompts: none "No parameters"
      mask help: Place copyright information at the top of every subsystem in design.
      mask Display:
      | NxtrConf = 'Nexteer Confidential';
      | 
      | sys = bdroot; %handle for the current model ("system")
      | first = get_param(sys,'Created');
      | first = first(end-3:end);  %year is last four digits
      | 
      | last = get_param(sys,'LastModifiedDate');
      | if isempty(last)
      |     last = datestr(now,'yyyy');
      | else
      |     last = last(end-3:end);
      | end
      | 
      | if strcmp(first,last)
      |     fprintf('%s -- Copyright %s Nexteer',NxtrConf,first)
      | else
      |     fprintf('%s -- %s%s- %s Nexteer',NxtrConf,char(169),first,last)
      | end
  Ivtr1Inactv_IF : If  RequirementInfo="{'linktype_rmi_doors' '0000bab3 (/E-STEER Core/SubSystem Specifications/Application Functions/SF049A Loss of Assist Manager)' '#SF049A_183' 'true' 'REQ:  SF049A_183' '' } %GIDa_1d0fb7e6_1c31_4e80_b36a_c03c6493b93e"  IfExpression=u1
  Ivtr1Sts_ELSE : Subsystem  RequirementInfo="{'linktype_rmi_doors' '0000bab3 (/E-STEER Core/SubSystem Specifications/Application Functions/SF049A Loss of Assist Manager)' '#SF049A_183' 'true' 'REQ:  SF049A_183' '' } %GIDa_bb509f56_fab0_4491_9374_c8286d7f8b29"  TreatAsAtomicUnit=on
      settings: RTWSystemCode=Inline
  Ivtr1Sts_THEN : Subsystem  RequirementInfo="{'linktype_rmi_doors' '0000bab3 (/E-STEER Core/SubSystem Specifications/Application Functions/SF049A Loss of Assist Manager)' '#SF049A_183' 'true' 'REQ:  SF049A_183' '' } %GIDa_1ef07b77_2ef9_4bc8_8364_62f92239dd9c"  TreatAsAtomicUnit=on
      settings: RTWSystemCode=Inline
  Ivtr2Inactv_IF : If  RequirementInfo="{'linktype_rmi_doors' '0000bab3 (/E-STEER Core/SubSystem Specifications/Application Functions/SF049A Loss of Assist Manager)' '#SF049A_183' 'true' 'REQ:  SF049A_183' '' } %GIDa_49badaa6_5497_4d2a_868f_8b14f223113a"  IfExpression=u1
  Ivtr2Sts_ELSE : Subsystem  RequirementInfo="{'linktype_rmi_doors' '0000bab3 (/E-STEER Core/SubSystem Specifications/Application Functions/SF049A Loss of Assist Manager)' '#SF049A_183' 'true' 'REQ:  SF049A_183' '' } %GIDa_3ba0abf9_881f_4bb2_8956_d482cda6ed77"  TreatAsAtomicUnit=on
      settings: RTWSystemCode=Inline
  Ivtr2Sts_THEN : Subsystem  RequirementInfo="{'linktype_rmi_doors' '0000bab3 (/E-STEER Core/SubSystem Specifications/Application Functions/SF049A Loss of Assist Manager)' '#SF049A_183' 'true' 'REQ:  SF049A_183' '' } %GIDa_ef66edbf_481c_40ba_884d_7aa7ea0834d3"  TreatAsAtomicUnit=on
      settings: RTWSystemCode=Inline
  IvtrIdptSig : Outport  RequirementInfo="{'linktype_rmi_doors' '0000bab3 (/E-STEER Core/SubSystem Specifications/Application Functions/SF049A Loss of Assist Manager)' '#SF049A_183' 'true' 'REQ:  SF049A_183' '' } %GIDa_1ffe7b96_2b91_4174_963d_04d74edc06f1"
  wires:
  " "/1 -> Add1/1
  " 1"/1 -> Add1/2
  Ivtr2Inactv_IF/1 -> Ivtr2Sts_THEN/Action
  Constant2/1 -> Ivtr2Sts_THEN/1(In1)
  Ivtr2Sts_THEN/1(Out1) -> " 1"/1
  Ivtr2Sts_ELSE/1(Out1) -> " 1"/2
  Ivtr2Inactv/1 -> Ivtr2Inactv_IF/1
  Ivtr1Inactv_IF/2 -> Ivtr1Sts_ELSE/Action
  Ivtr1Inactv_IF/1 -> Ivtr1Sts_THEN/Action
  Constant6/1 -> Ivtr1Sts_ELSE/1(In1)
  Ivtr1Sts_ELSE/1(Out1) -> " "/2
  Ivtr1Inactv/1 -> Ivtr1Inactv_IF/1
  Constant1/1 -> Ivtr2Sts_ELSE/1(In1)
  Ivtr2Inactv_IF/2 -> Ivtr2Sts_ELSE/Action
  Constant4/1 -> Ivtr1Sts_THEN/1(In1)
  Ivtr1Sts_THEN/1(Out2) -> " "/1
  Add1/1 -> IvtrIdptSig/1

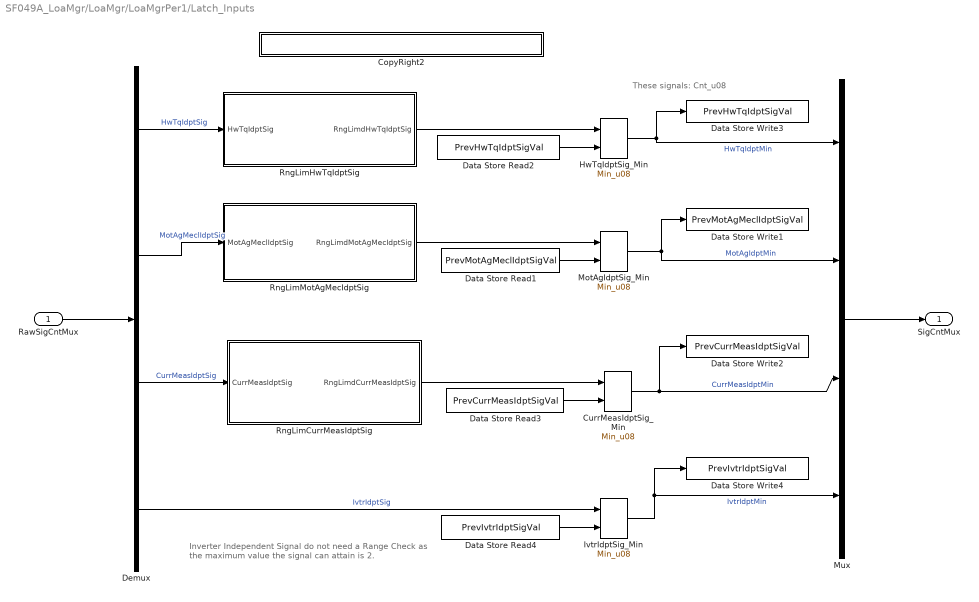
== system SF049A_LoaMgr/LoaMgr/LoaMgrPer1/Latch_Inputs ==
  note: Inverter Independent Signal do not need a Range Check
      | as the maximum value the signal can attain is 2.
  note: These signals: Cnt_u08
  RawSigCntMux : Inport  RequirementInfo={} %GIDa_570c76ce_5bdc_4ab1_b26d_82258c3ad709
  CopyRight2 : Subsystem  Description=|  mask(Copyright Information){none=on}
      | Copyright info block.                                               
      |                                                                     
      | Place copyright information at the top of every subsystem in design.
      mask prompts: none "No parameters"
      mask help: Place copyright information at the top of every subsystem in design.
      mask Display:
      | NxtrConf = 'Nexteer Confidential';
      | 
      | sys = bdroot; %handle for the current model ("system")
      | first = get_param(sys,'Created');
      | first = first(end-3:end);  %year is last four digits
      | 
      | last = get_param(sys,'LastModifiedDate');
      | if isempty(last)
      |     last = datestr(now,'yyyy');
      | else
      |     last = last(end-3:end);
      | end
      | 
      | if strcmp(first,last)
      |     fprintf('%s -- Copyright %s Nexteer',NxtrConf,first)
      | else
      |     fprintf('%s -- %s%s- %s Nexteer',NxtrConf,char(169),first,last)
      | end
  CurrMeasIdptSig_Min : NxtrMin/Min_u08  SFunctionSpec="uint8 y1 = Min_u08( uint8 u1,  uint8 u2)"  ShowSpec=off
      settings: AttributesFormatString=%<Name>
  Data Store Read1 : DataStoreRead  DataStoreName=PrevMotAgMeclIdptSigVal
  Data Store Read2 : DataStoreRead  DataStoreName=PrevHwTqIdptSigVal
  Data Store Read3 : DataStoreRead  DataStoreName=PrevCurrMeasIdptSigVal
  Data Store Read4 : DataStoreRead  DataStoreName=PrevIvtrIdptSigVal
  Data Store Write1 : DataStoreWrite  DataStoreName=PrevMotAgMeclIdptSigVal
  Data Store Write2 : DataStoreWrite  DataStoreName=PrevCurrMeasIdptSigVal
  Data Store Write3 : DataStoreWrite  DataStoreName=PrevHwTqIdptSigVal
  Data Store Write4 : DataStoreWrite  DataStoreName=PrevIvtrIdptSigVal
  Demux : Demux
  HwTqIdptSig_Min : NxtrMin/Min_u08  SFunctionSpec="uint8 y1 = Min_u08( uint8 u1,  uint8 u2)"  ShowSpec=off
      settings: AttributesFormatString=%<Name>
  IvtrIdptSig_Min : NxtrMin/Min_u08  SFunctionSpec="uint8 y1 = Min_u08( uint8 u1,  uint8 u2)"  ShowSpec=off
      settings: AttributesFormatString=%<Name>
  MotAgIdptSig_Min : NxtrMin/Min_u08  SFunctionSpec="uint8 y1 = Min_u08( uint8 u1,  uint8 u2)"  ShowSpec=off
      settings: AttributesFormatString=%<Name>
  Mux : Mux
  RngLimCurrMeasIdptSig : Subsystem  RequirementInfo="{'linktype_rmi_doors' '0000bab3 (/E-STEER Core/SubSystem Specifications/Application Functions/SF049A Loss of Assist Manager)' '#SF049A_188' 'true' 'REQ:  SF049A_188' '' } %GIDa_999e66fd_079b_47d1_9e58_0c4ad5ab9491"
  RngLimHwTqIdptSig : Subsystem  RequirementInfo="{'linktype_rmi_doors' '0000bab3 (/E-STEER Core/SubSystem Specifications/Application Functions/SF049A Loss of Assist Manager)' '#SF049A_186' 'true' 'REQ:  SF049A_186' '' } %GIDa_2d40f268_9dd8_45c1_9fdf_d84f9d64878c"
  RngLimMotAgMecIdptSig : Subsystem  RequirementInfo="{'linktype_rmi_doors' '0000bab3 (/E-STEER Core/SubSystem Specifications/Application Functions/SF049A Loss of Assist Manager)' '#SF049A_187' 'true' 'REQ:  SF049A_187' '' } %GIDa_f596fe09_953c_4e69_95f6_8719f0f87990"
  SigCntMux : Outport  RequirementInfo={} %GIDa_5bf316b9_153e_4737_96bd_43ea582c932b
  wires:
  Demux/2 -> RngLimMotAgMecIdptSig/1(MotAgMeclIdptSig)  "MotAgMeclIdptSig"
  HwTqIdptSig_Min/1 -> Mux/1, Data Store Write3/1  "HwTqIdptMin"
  CurrMeasIdptSig_Min/1 -> Mux/3, Data Store Write2/1  "CurrMeasIdptMin"
  Demux/4 -> IvtrIdptSig_Min/1  "IvtrIdptSig"
  IvtrIdptSig_Min/1 -> Data Store Write4/1, Mux/4  "IvtrIdptMin"
  Demux/3 -> RngLimCurrMeasIdptSig/1(CurrMeasIdptSig)  "CurrMeasIdptSig"
  Mux/1 -> SigCntMux/1
  RawSigCntMux/1 -> Demux/1
  Demux/1 -> RngLimHwTqIdptSig/1(HwTqIdptSig)  "HwTqIdptSig"
  RngLimMotAgMecIdptSig/1(RngLimdMotAgMecIdptSig) -> MotAgIdptSig_Min/1
  RngLimHwTqIdptSig/1(RngLimdHwTqIdptSig) -> HwTqIdptSig_Min/1
  MotAgIdptSig_Min/1 -> Mux/2, Data Store Write1/1  "MotAgIdptMin"
  Data Store Read1/1 -> MotAgIdptSig_Min/2
  Data Store Read4/1 -> IvtrIdptSig_Min/2
  Data Store Read2/1 -> HwTqIdptSig_Min/2
  RngLimCurrMeasIdptSig/1(RngLimdCurrMeasIdptSig) -> CurrMeasIdptSig_Min/1
  Data Store Read3/1 -> CurrMeasIdptSig_Min/2

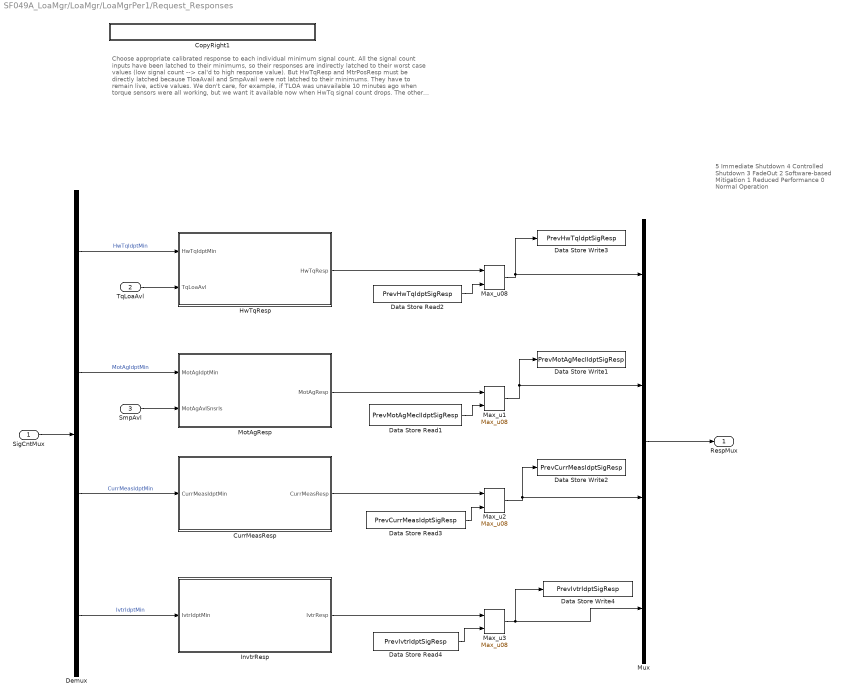
== system SF049A_LoaMgr/LoaMgr/LoaMgrPer1/Request_Responses ==
  note: Choose appropriate calibrated response to each individual minimum signal count.  All the signal count inputs have been latched to their minimums,
      | so their responses are indirectly latched to their worst case values (low signal count --> cal'd to high response value).  But HwTqResp and
      | MtrPosResp must be directly latched because TloaAvail and SmpAvail were not latched to their minimums.  They have to remain live, active values.
      | We don't care, for example, if TLOA was unavailable 10 minutes ago when torque sensors were all working, but we want it available now when
      | HwTq signal count drops.
      |
      | The other two (MotCurrResp and IvtrResp) are being latched as defensive programming against inappropriate calibration values.  Peer review group
      | had concerns about a scenerio like this:  (IdptSig=2, Resp=Normal) and (IdptSig=1, Resp=SwMtgtn) and (IdptSig=0, Resp=Normal).
  note: 5 Immediate Shutdown
      | 4 Controlled Shutdown
      | 3 FadeOut
      | 2 Software-based Mitigation
      | 1 Reduced Performance
      | 0 Normal Operation
  SigCntMux : Inport
  TqLoaAvl : Inport  RequirementInfo={} %GIDa_67da4e6f_783e_4b7f_b2da_bafe95c201fd  Port=2
  SmpAvl : Inport  RequirementInfo={} %GIDa_69e486c7_ff85_439f_a16b_5dc177bb9ace  Port=3
  CopyRight1 : Subsystem  Description=|  mask(Copyright Information){none=on}
      | Copyright info block.                                               
      |                                                                     
      | Place copyright information at the top of every subsystem in design.
      mask prompts: none "No parameters"
      mask help: Place copyright information at the top of every subsystem in design.
      mask Display:
      | NxtrConf = 'Nexteer Confidential';
      | 
      | sys = bdroot; %handle for the current model ("system")
      | first = get_param(sys,'Created');
      | first = first(end-3:end);  %year is last four digits
      | 
      | last = get_param(sys,'LastModifiedDate');
      | if isempty(last)
      |     last = datestr(now,'yyyy');
      | else
      |     last = last(end-3:end);
      | end
      | 
      | if strcmp(first,last)
      |     fprintf('%s -- Copyright %s Nexteer',NxtrConf,first)
      | else
      |     fprintf('%s -- %s%s- %s Nexteer',NxtrConf,char(169),first,last)
      | end
  CurrMeasResp : Subsystem
  Data Store Read1 : DataStoreRead  RequirementInfo="{'linktype_rmi_doors' '0000bab3 (/E-STEER Core/SubSystem Specifications/Application Functions/SF049A Loss of Assist Manager)' '#SF049A_176' 'true' 'REQ:  SF049A_176' '' } %GIDa_d5e80c01_4438_4861_b095_cff7a06fcce6"  DataStoreName=PrevMotAgMeclIdptSigResp
  Data Store Read2 : DataStoreRead  RequirementInfo="{'linktype_rmi_doors' '0000bab3 (/E-STEER Core/SubSystem Specifications/Application Functions/SF049A Loss of Assist Manager)' '#SF049A_175' 'true' 'REQ:  SF049A_175' '' } %GIDa_73fa6eca_3065_4e69_8a70_8a244e0f93c6"  DataStoreName=PrevHwTqIdptSigResp
  Data Store Read3 : DataStoreRead  RequirementInfo="{'linktype_rmi_doors' '0000bab3 (/E-STEER Core/SubSystem Specifications/Application Functions/SF049A Loss of Assist Manager)' '#SF049A_177' 'true' 'REQ:  SF049A_177' '' } %GIDa_1294041b_422f_4480_b8e7_16eab3642230"  DataStoreName=PrevCurrMeasIdptSigResp
  Data Store Read4 : DataStoreRead  RequirementInfo="{'linktype_rmi_doors' '0000bab3 (/E-STEER Core/SubSystem Specifications/Application Functions/SF049A Loss of Assist Manager)' '#SF049A_178' 'true' 'REQ:  SF049A_178' '' } %GIDa_19366f79_04b6_40aa_baeb_0d5ed61e154b"  DataStoreName=PrevIvtrIdptSigResp
  Data Store Write1 : DataStoreWrite  RequirementInfo="{'linktype_rmi_doors' '0000bab3 (/E-STEER Core/SubSystem Specifications/Application Functions/SF049A Loss of Assist Manager)' '#SF049A_176' 'true' 'REQ:  SF049A_176' '' } %GIDa_32a932cd_02cb_42c7_b0fb_9fdd187e6814"  DataStoreName=PrevMotAgMeclIdptSigResp
  Data Store Write2 : DataStoreWrite  RequirementInfo="{'linktype_rmi_doors' '0000bab3 (/E-STEER Core/SubSystem Specifications/Application Functions/SF049A Loss of Assist Manager)' '#SF049A_177' 'true' 'REQ:  SF049A_177' '' } %GIDa_3a10439b_5464_4f3c_bdbe_f45764853848"  DataStoreName=PrevCurrMeasIdptSigResp
  Data Store Write3 : DataStoreWrite  RequirementInfo="{'linktype_rmi_doors' '0000bab3 (/E-STEER Core/SubSystem Specifications/Application Functions/SF049A Loss of Assist Manager)' '#SF049A_175' 'true' 'REQ:  SF049A_175' '' } %GIDa_837e576b_0fbd_4152_95b8_d68d34ed0829"  DataStoreName=PrevHwTqIdptSigResp
  Data Store Write4 : DataStoreWrite  RequirementInfo="{'linktype_rmi_doors' '0000bab3 (/E-STEER Core/SubSystem Specifications/Application Functions/SF049A Loss of Assist Manager)' '#SF049A_178' 'true' 'REQ:  SF049A_178' '' } %GIDa_72f63d78_8ac9_4799_b250_7f073763e93c"  DataStoreName=PrevIvtrIdptSigResp
  Demux : Demux
  HwTqResp : Subsystem
  InvtrResp : Subsystem
  Max_u08 : NxtrMax/Max_u08  RequirementInfo="{'linktype_rmi_doors' '0000bab3 (/E-STEER Core/SubSystem Specifications/Application Functions/SF049A Loss of Assist Manager)' '#SF049A_175' 'true' 'REQ:  SF049A_175' '' } %GIDa_0b74d1c9_9f8c_415e_9ecd_2ee161ecdea1"  SFunctionSpec="uint8 y1 = Max_u08( uint8 u1,  uint8 u2)"
      settings: AttributesFormatString=%<Name>
  Max_u1 : NxtrMax/Max_u08  RequirementInfo="{'linktype_rmi_doors' '0000bab3 (/E-STEER Core/SubSystem Specifications/Application Functions/SF049A Loss of Assist Manager)' '#SF049A_176' 'true' 'REQ:  SF049A_176' '' } %GIDa_0a8fc13e_1cdd_4713_9663_6ccd78ac61a5"  SFunctionSpec="uint8 y1 = Max_u08( uint8 u1,  uint8 u2)"
      settings: AttributesFormatString=%<Name>
  Max_u2 : NxtrMax/Max_u08  RequirementInfo="{'linktype_rmi_doors' '0000bab3 (/E-STEER Core/SubSystem Specifications/Application Functions/SF049A Loss of Assist Manager)' '#SF049A_177' 'true' 'REQ:  SF049A_177' '' } %GIDa_15c2933b_3ee1_464e_9187_c8c3c4498ff8"  SFunctionSpec="uint8 y1 = Max_u08( uint8 u1,  uint8 u2)"
      settings: AttributesFormatString=%<Name>
  Max_u3 : NxtrMax/Max_u08  RequirementInfo="{'linktype_rmi_doors' '0000bab3 (/E-STEER Core/SubSystem Specifications/Application Functions/SF049A Loss of Assist Manager)' '#SF049A_178' 'true' 'REQ:  SF049A_178' '' } %GIDa_94d9758b_79b1_4700_bad7_ebcda6c03edc"  SFunctionSpec="uint8 y1 = Max_u08( uint8 u1,  uint8 u2)"
      settings: AttributesFormatString=%<Name>
  MotAgResp : Subsystem
  Mux : Mux
  RespMux : Outport
  wires:
  Demux/1 -> HwTqResp/1(HwTqIdptMin)  "HwTqIdptMin"
  Demux/3 -> CurrMeasResp/1(CurrMeasIdptMin)  "CurrMeasIdptMin"
  Demux/4 -> InvtrResp/1(IvtrIdptMin)  "IvtrIdptMin"
  Demux/2 -> MotAgResp/1(MotAgIdptMin)  "MotAgIdptMin"
  SigCntMux/1 -> Demux/1
  Mux/1 -> RespMux/1
  TqLoaAvl/1 -> HwTqResp/2(TqLoaAvl)
  SmpAvl/1 -> MotAgResp/2(MotAgAvlSnsrls)
  HwTqResp/1(HwTqResp) -> Max_u08/1
  Max_u08/1 -> Data Store Write3/1, Mux/1
  MotAgResp/1(MotAgResp) -> Max_u1/1
  CurrMeasResp/1(CurrMeasResp) -> Max_u2/1
  Max_u2/1 -> Data Store Write2/1, Mux/3
  InvtrResp/1(IvtrResp) -> Max_u3/1
  Max_u3/1 -> Data Store Write4/1, Mux/4
  Data Store Read2/1 -> Max_u08/2
  Max_u1/1 -> Data Store Write1/1, Mux/2
  Data Store Read1/1 -> Max_u1/2
  Data Store Read3/1 -> Max_u2/2
  Data Store Read4/1 -> Max_u3/2
